simulink model "test_mosfet_dynamic"  (R2021b)
settings: Solver=VariableStepAuto  StartTime=0.0  StopTime=0.1  RelTol=1e-3
libraries: fl_lib x17, nesl_utility x12, ee_lib x5, simulink x1
settings Model: PauseTimes=0.1  Creator=khduh  LastModifiedBy=user
settings DataIOCC: SaveState=on
settings SimscapeCC: SimscapeLogType=all  SimscapeLogLimitData=off

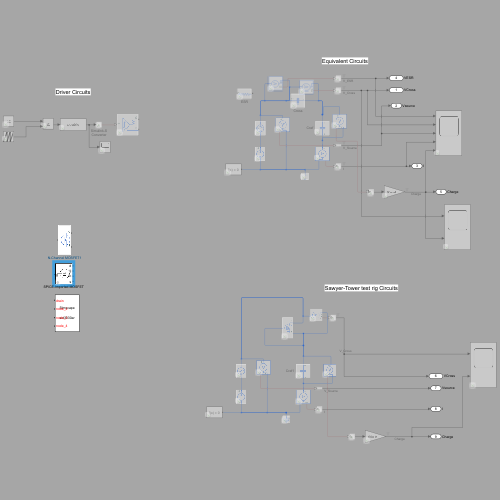
[thumbnail: Simulink's stored preview of the top-level diagram]
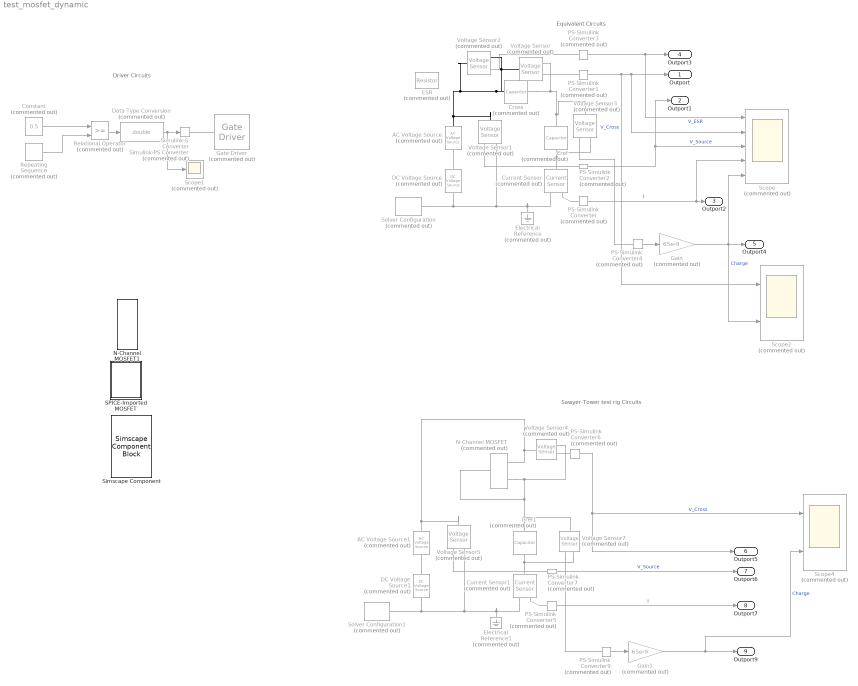
== system test_mosfet_dynamic ==
  note: Driver Circuits
  note: Equivalent Circuits
  note: Sawyer-Tower test rig Circuits
  AC Voltage Source : fl_lib/Electrical/Electrical Sources/AC Voltage Source  Commented=on  amp=50 V  shift=0 deg  frequency=60 Hz  omega=0 rad/s
  AC Voltage Source1 : fl_lib/Electrical/Electrical Sources/AC Voltage Source  Commented=on  amp=50 V  shift=0 deg  frequency=60 Hz  omega=0 rad/s
  Constant : Constant  Commented=on  Value=0.5
  Cref : fl_lib/Electrical/Electrical Elements/Capacitor  Commented=on  c=65e-9 F  r=1e-6 Ohm  g=0 1/Ohm  i_specify=off  i_priority=None  i=0 A  i_nominal_specify=off  i_nominal_unit=A  i_nominal_value=1  v_specify=off  v_priority=None  v=0 V  v_nominal_specify=off  v_nominal_unit=V  v_nominal_value=1  vc_specify=off  vc_priority=High  vc=0 V  vc_nominal_specify=off  vc_nominal_unit=V  vc_nominal_value=1
  Cref1 : fl_lib/Electrical/Electrical Elements/Capacitor  Commented=on  c=65e-9 F  r=1e-6 Ohm  g=0 1/Ohm  i_specify=off  i_priority=None  i=0 A  i_nominal_specify=off  i_nominal_unit=A  i_nominal_value=1  v_specify=off  v_priority=None  v=0 V  v_nominal_specify=off  v_nominal_unit=V  v_nominal_value=1  vc_specify=off  vc_priority=High  vc=0 V  vc_nominal_specify=off  vc_nominal_unit=V  vc_nominal_value=1
  Cross : fl_lib/Electrical/Electrical Elements/Capacitor  Commented=on  c=89e-9 F  r=1e-6 Ohm  g=0 1/Ohm  i_specify=off  i_priority=None  i=0 A  i_nominal_specify=off  i_nominal_unit=A  i_nominal_value=1  v_specify=off  v_priority=None  v=0 V  v_nominal_specify=off  v_nominal_unit=V  v_nominal_value=1  vc_specify=off  vc_priority=High  vc=0 V  vc_nominal_specify=off  vc_nominal_unit=V  vc_nominal_value=1
  Current Sensor : fl_lib/Electrical/Electrical Sensors/Current Sensor  Commented=on
  Current Sensor1 : fl_lib/Electrical/Electrical Sensors/Current Sensor  Commented=on
  DC Voltage Source : ee_lib/Additional Components/SPICE Sources/DC Voltage Source  Commented=on  DC=100 V
  DC Voltage Source1 : ee_lib/Additional Components/SPICE Sources/DC Voltage Source  Commented=on  DC=500 V
  Data Type Conversion : DataTypeConversion  Commented=on  OutDataTypeStr=double
  ESR : fl_lib/Electrical/Electrical Elements/Resistor  Commented=on  R=58.5e3 Ohm  i_specify=off  i_priority=None  i=0 A  i_nominal_specify=off  i_nominal_unit=A  i_nominal_value=1  v_specify=off  v_priority=None  v=0 V  v_nominal_specify=off  v_nominal_unit=V  v_nominal_value=1
  Electrical Reference : fl_lib/Electrical/Electrical Elements/Electrical Reference  Commented=on
  Electrical Reference1 : fl_lib/Electrical/Electrical Elements/Electrical Reference  Commented=on
  Gain : Gain  Commented=on  Gain=65e-9
  Gain1 : Gain  Commented=on  Gain=65e-9
  Gate Driver : ee_lib/Semiconductors & Converters/Gate Driver  Commented=on  uHighValue=0.7  uLowValue=0.3  vHigh=4 V  vLow=0 V  tHigh=50 ns  tLow=50 ns  parameterization=1  rHigh=2 Ohm  rLow=2 Ohm  tRise=20 ns  tFall=20 ns  cLoad=10 nF  enable_faults=0  t_fault=1 s  fault_type=1  ZonTime_specify=off  ZonTime_priority=None  ZonTime=0 s  ZoffTime_specify=off  ZoffTime_priority=None  ZoffTime=0 s  uHigh=2.0 V  uLow=0.8 V
      settings: SourceProductBaseCode=PS  InternalSimscapePortConfiguration="{\"Bottom\":[],\"Left\":[{\"id\":\"u\",\"label\":\"u\",\"type\":\"input\"}],\"Right\":[{\"id\":\"G\",\"label\":\"G\",\"type\":\"foundation.electrical.electrical\"},{\"id\":\"S\",\"label\":\"S\",\"type\":\"foundation.electrical.electrical\"}],\"Top\":[]}"
  N-Channel MOSFET : ee_lib/Semiconductors & Converters/N-Channel MOSFET  Commented=on  paramTerminal=ee.enum.mosfet.numberOfTerminals.three  parameterization=ee.enum.mosfet.parameterization.datasheet  Beta=5.0 A/V^2  Rds=0.025 Ohm  Id=6.0 A  Vgs=10 V  Vth=1.7 V  Vth0=1.7 V  lam=0 1/V  gamma_vth=0.5 V^(1/2)  phib=0.5 V  Vth1=1.9071 V  Vbs1=-1 V  Vth2=2.066 V  Vbs2=-2 V  Tmeas=25 degC  Vgs_vec=[-.5, 2, 3, 4, 5] V  Vds_vec=[0, 2, 4, 8, 12, 16, 20] V  Vbs_vec=[0, -4, -6, -12] V  T_vec=[25, 125] degC  Vth_vec=[.4, 1.2, 1.4, 1.45] V  Vth_mat=[.4, .35; 1.2, 1.15; 1.4, 1.35; 1.45, 1.4] V  Ids_mat=[0, 0, 0, 0, 0, 0, 0; 0, .003, .0038, .0043, .0046, .0048, .0049; 0, .0055, .008, .009, .0095, .01, .0101; 0, .0115, .016, .018, .019, .0195, .02; 0, .0152, .0225, .0265, .028, .0295, .03] A  Ids_mat0=[0, 0, 0, 0, 0, 0, 0; 0, .003, .0038, .0043, .0046, .0048, .0049; 0, .0055, .008, .009, .0095, .01, .0101; 0, .0115, .016, .018, .019, .0195, .02; 0, .0152, .0225, .0265, .028, .0295, .03] A  Ids_mat_3D=zeros(5, 7, 2) A  Ids_mat_3D0=zeros(5, 7, 2) A  IV_table_symmetry=ee.enum.mosfet.symmetricNIV.no  RS=0.0001 Ohm  RD=0.01 Ohm  RB=0.001 Ohm  C_param=ee.enum.mosfet.capacitanceParam.fixedciss  C_GS=270 pF  C_GD=80 pF  C_DS=0 pF  C_iss=1526 pF  C_rss=42 pF  C_oss=89 pF  charge_linearity_param=ee.enum.mosfet.cgdLinearity.constant  C_OX=200 pF  V_C_OX=-0.5 V  charge_linearity_param_vgb=ee.enum.mosfet.cgbLinearity.instantly  C_iss_vec=[720, 700, 590, 470, 390, 310] pF  C_rss_vec=[450, 400, 300, 190, 95, 55] pF  C_oss_vec=[900, 810, 690, 420, 270, 170] pF  C_GS_vec=[270, 300, 290, 280, 295, 255] pF  C_GD_vec=[450, 400, 300, 190, 95, 55] pF  C_DS_vec=[450, 410, 390, 230, 175, 115] pF  C_Vds_vec=[.1, .3, 1, 3, 10, 30] V  V_GS_for_cap_data=0 V  Di_param=ee.enum.mosfet.diodeParam.no  IsDiode=0 A  Vbi=0.6 V  n=1  Cj0Diode=0 pF  TT=50e-9 s  Tmeas_dio=25 degC  TableTypeNoT=ee.enum.mosfet.tableType.IfMat  TableType=ee.enum.diode.tableType.IfMat  IfVec=[.07, .12, .19, 1.75, 4.24, 7.32, 11.2] A  IfMat=[.07, .12, .19, 1.75, 4.24, 7.32, 11.2; .16, .3, .72, 2.14, 4.02, 6.35, 9.12] A  VfVecV=[.9, 1.15, 1.25, 1.5, 1.75, 2.17, 2.6, 2.85] V  VfMatV=[.9, 1.15, 1.25, 1.5, 1.75, 2.17, 2.6, 2.85; .58, .68, .75, 1.1, 1.38, 1.77, 2.27, 2.7] V  TjVec=[25, 125] degC  VfVec=[.5, .7, .9, 1.3, 1.7, 2.1, 2.5] V  IfVecV=[.1, .2, .5, 1, 2, 4, 7, 10] A  prmDatasheet=ee.enum.temperatureParameterization.none  prmEquCoeff=ee.enum.temperatureParameterization.none  dVth_dT=-6 mV/K  dVth0_dT=-6 mV/K  Rds_T2=0.037 Ohm  BEXDatasheet=-1.5  BEXEquCoeff=-1.5  etaisDatasheet=3  etaisEquCoeff=3  Tmeas2=125 degC  etaisTabulated=3  TdeviceDatasheet=25 degC  TdeviceEquCoeff=25 degC  TdeviceTabulated=25 degC  thermal_network_parameterization=ee.enum.thermalNetworkTopology.junctionCase  Rth=[0, 10] K/W  Rth_Cauer=[1, 3, 10] K/W  Rth_Foster=[4, 6] K/W  thermal_mass_parameterization=ee.enum.thermalNetwork.timeconstant  thermal_mass=[0, 1] J/K  thermal_mass_Cauer=[.1, .3, 1] J/K  thermal_mass_Foster=[1.5, 3] J/K  thermal_time_constant=[0, 10] s  thermal_time_constant_Cauer=[1, 3, 10] s  thermal_time_constant_Foster=[6, 18] s  thermal_mass_initial_temperatures=[25, 25] degC  thermal_mass_initial_temperatures_Cauer=[25, 25, 25] degC  steadyState_Foster=simscape.enum.onoff.on  Tvec_initial_Foster=[25, 25, 25, 25] degC  betaref=18 A/V^2  Vfbref=-1.1 V  gamma=3.5 V^(1/2)  phib2ref=1 V  thesatref=0.4 1/V  alpha=0  Vp=5e-2 V  thesrref=0 1/V  m=8  Tref=25 degC  Rsref=2e-3 Ohm  Rdref=0.17 Ohm  Rgref=8.4 Ohm  Rbref=2e-3 Ohm  Cox=1500 pF  Cgso=100 pF  Cgdo=14 pF  Isref=5.2e-13 A  Cj0=480 pF  Tprm=1  etabet=1.3  Stvfb=5e-4 V/K  Stphib=-8.5e-4 V/K  etasat=1.04  etasr=0.65  etar=0.95  etais=3  Tsim=25 degC  T0=[25, 25] degC  T0_Cauer=[25, 25, 25] degC
  N-Channel MOSFET1 : ee_lib/Semiconductors & Converters/N-Channel MOSFET  paramTerminal=ee.enum.mosfet.numberOfTerminals.three  parameterization=ee.enum.mosfet.parameterization.datasheet  Beta=5.0 A/V^2  Rds=0.025 Ohm  Id=6.0 A  Vgs=10 V  Vth=1.7 V  Vth0=1.7 V  lam=0 1/V  gamma_vth=0.5 V^(1/2)  phib=0.5 V  Vth1=1.9071 V  Vbs1=-1 V  Vth2=2.066 V  Vbs2=-2 V  Tmeas=25 degC  Vgs_vec=[-.5, 2, 3, 4, 5] V  Vds_vec=[0, 2, 4, 8, 12, 16, 20] V  Vbs_vec=[0, -4, -6, -12] V  T_vec=[25, 125] degC  Vth_vec=[.4, 1.2, 1.4, 1.45] V  Vth_mat=[.4, .35; 1.2, 1.15; 1.4, 1.35; 1.45, 1.4] V  Ids_mat=[0, 0, 0, 0, 0, 0, 0; 0, .003, .0038, .0043, .0046, .0048, .0049; 0, .0055, .008, .009, .0095, .01, .0101; 0, .0115, .016, .018, .019, .0195, .02; 0, .0152, .0225, .0265, .028, .0295, .03] A  Ids_mat0=[0, 0, 0, 0, 0, 0, 0; 0, .003, .0038, .0043, .0046, .0048, .0049; 0, .0055, .008, .009, .0095, .01, .0101; 0, .0115, .016, .018, .019, .0195, .02; 0, .0152, .0225, .0265, .028, .0295, .03] A  Ids_mat_3D=zeros(5, 7, 2) A  Ids_mat_3D0=zeros(5, 7, 2) A  IV_table_symmetry=ee.enum.mosfet.symmetricNIV.no  RS=0.0001 Ohm  RD=0.01 Ohm  RB=0.001 Ohm  C_param=ee.enum.mosfet.capacitanceParam.fixedciss  C_GS=270 pF  C_GD=80 pF  C_DS=0 pF  C_iss=350 pF  C_rss=80 pF  C_oss=0 pF  charge_linearity_param=ee.enum.mosfet.cgdLinearity.constant  C_OX=200 pF  V_C_OX=-0.5 V  charge_linearity_param_vgb=ee.enum.mosfet.cgbLinearity.instantly  C_iss_vec=[720, 700, 590, 470, 390, 310] pF  C_rss_vec=[450, 400, 300, 190, 95, 55] pF  C_oss_vec=[900, 810, 690, 420, 270, 170] pF  C_GS_vec=[270, 300, 290, 280, 295, 255] pF  C_GD_vec=[450, 400, 300, 190, 95, 55] pF  C_DS_vec=[450, 410, 390, 230, 175, 115] pF  C_Vds_vec=[.1, .3, 1, 3, 10, 30] V  V_GS_for_cap_data=0 V  Di_param=ee.enum.mosfet.diodeParam.no  IsDiode=0 A  Vbi=0.6 V  n=1  Cj0Diode=0 pF  TT=50e-9 s  Tmeas_dio=25 degC  TableTypeNoT=ee.enum.mosfet.tableType.IfMat  TableType=ee.enum.diode.tableType.IfMat  IfVec=[.07, .12, .19, 1.75, 4.24, 7.32, 11.2] A  IfMat=[.07, .12, .19, 1.75, 4.24, 7.32, 11.2; .16, .3, .72, 2.14, 4.02, 6.35, 9.12] A  VfVecV=[.9, 1.15, 1.25, 1.5, 1.75, 2.17, 2.6, 2.85] V  VfMatV=[.9, 1.15, 1.25, 1.5, 1.75, 2.17, 2.6, 2.85; .58, .68, .75, 1.1, 1.38, 1.77, 2.27, 2.7] V  TjVec=[25, 125] degC  VfVec=[.5, .7, .9, 1.3, 1.7, 2.1, 2.5] V  IfVecV=[.1, .2, .5, 1, 2, 4, 7, 10] A  prmDatasheet=ee.enum.temperatureParameterization.none  prmEquCoeff=ee.enum.temperatureParameterization.none  dVth_dT=-6 mV/K  dVth0_dT=-6 mV/K  Rds_T2=0.037 Ohm  BEXDatasheet=-1.5  BEXEquCoeff=-1.5  etaisDatasheet=3  etaisEquCoeff=3  Tmeas2=125 degC  etaisTabulated=3  TdeviceDatasheet=25 degC  TdeviceEquCoeff=25 degC  TdeviceTabulated=25 degC  thermal_network_parameterization=ee.enum.thermalNetworkTopology.junctionCase  Rth=[0, 10] K/W  Rth_Cauer=[1, 3, 10] K/W  Rth_Foster=[4, 6] K/W  thermal_mass_parameterization=ee.enum.thermalNetwork.timeconstant  thermal_mass=[0, 1] J/K  thermal_mass_Cauer=[.1, .3, 1] J/K  thermal_mass_Foster=[1.5, 3] J/K  thermal_time_constant=[0, 10] s  thermal_time_constant_Cauer=[1, 3, 10] s  thermal_time_constant_Foster=[6, 18] s  thermal_mass_initial_temperatures=[25, 25] degC  thermal_mass_initial_temperatures_Cauer=[25, 25, 25] degC  steadyState_Foster=simscape.enum.onoff.on  Tvec_initial_Foster=[25, 25, 25, 25] degC  betaref=18 A/V^2  Vfbref=-1.1 V  gamma=3.5 V^(1/2)  phib2ref=1 V  thesatref=0.4 1/V  alpha=0  Vp=5e-2 V  thesrref=0 1/V  m=8  Tref=25 degC  Rsref=2e-3 Ohm  Rdref=0.17 Ohm  Rgref=8.4 Ohm  Rbref=2e-3 Ohm  Cox=1500 pF  Cgso=100 pF  Cgdo=14 pF  Isref=5.2e-13 A  Cj0=480 pF  Tprm=1  etabet=1.3  Stvfb=5e-4 V/K  Stphib=-8.5e-4 V/K  etasat=1.04  etasr=0.65  etar=0.95  etais=3  Tsim=25 degC  T0=[25, 25] degC  T0_Cauer=[25, 25, 25] degC
  PS-Simulink Converter{,1..7,9} (9 alike) : nesl_utility/PS-Simulink Converter  Commented=on  PhysicalDomain=network_engine_domain  SubClassName=ps_output  LeftPortType=input  RightPortType=output  PseudoPeriodic=off  Frequencies=[]  Unit=inherit  AffineConversion=off
      settings: SourceProductBaseCode=PW,SS
  Relational Operator : RelationalOperator  Commented=on  OutDataTypeStr=boolean  RndMeth=Simplest
  Repeating Sequence : simulink/Sources/Repeating Sequence  Commented=on  rep_seq_t=[0 100e-6]  rep_seq_y=[0 1]
  SPICE-Imported MOSFET : Subsystem  mask(SPICE-Imported MOSFET){SeriesChoice=Infineon OptiMOS6 40V, DeviceOptiMOS40V=IAUC120N04S6N009, DeviceOptiMOS60V=IPB120N06S4_H1, DeviceOptiMOS80V=IAUT300N08S5N012, DeviceOptiMOS120V=IPB100N12S3_05}
      mask prompts: SeriesChoice "Series"; DeviceOptiMOS40V "Device"; DeviceOptiMOS60V "Device"; DeviceOptiMOS80V "Device"; DeviceOptiMOS120V "Device"
      mask help: MOSFET model converted from SPICE.<br/> <br/> To view information pertaining to this device model, see the <a href="matlab: ee.internal.spice.openAndGoToLine('Infineon-OptiMOS6_40V-SimulationModels-v02_00-EN.lib','IAUC120N04S6N009')">originating SPICE file</a>.
      mask init:
      | ee.internal.spice.maskCallbackMOSFETs(gcb)
      settings: CopyFcn=set_param(gcb,'LinkStatus','none');
      mask Help: web(nesl_help(gcbh))
      mask TypeOptions SeriesChoice: Infineon OptiMOS6 40V | Infineon OptiMOS4 60V | Infineon OptiMOS5 80V | Infineon OptiMOST 120V
      mask Callback SeriesChoice:
      | %Run mask initialization to update the block help
      | ee.internal.spice.maskCallbackMOSFETs(gcb)
      mask TypeOptions DeviceOptiMOS40V: IAUC120N04S6N009 | IAUC120N04S6N010 | IAUC120N04S6N013 | IAUC100N04S6N015 | IAUC100N04S6N022 | IAUC100N04S6N028 | IAUC80N04S6N036 | IAUC60N04S6N044 | IAUC120N04S6L008 | IAUC120N04S6L009 | IAUC120N04S6L012 | IAUC100N04S6L014 | IAUC100N04S6L020 | IAUC100N04S6L025 | IAUC80N04S6L032 | IAUC60N04S6L039
      mask Callback DeviceOptiMOS40V:
      | %Run mask initialization to update the block help
      | ee.internal.spice.maskCallbackMOSFETs(gcb)
      mask TypeOptions DeviceOptiMOS60V: IPB180N06S4_H1 | IPB120N06S4_H1 | IPI120N06S4_H1 | IPP120N06S4_H1 | IPB120N06S4_02 | IPI120N06S4_02 | IPP120N06S4_02 | IPB120N06S4_03 | IPI120N06S4_03 | IPP120N06S4_03 | IPB90N06S4_04 | IPD90N06S4_04 | IPD100N06S4_03 | IPI90N06S4_04 | IPP90N06S4_04 | IPB80N06S4_05 | IPD90N06S4_05 | IPI80N06S4_05 | IPP80N06S4_05 | IPB80N06S4_07 | IPD90N06S4_07 | IPI80N06S4_07 | IPP80N06S4_07 | IPB45N06S4_09 | IPD50N06S4_09 | IPI45N06S4_09 | IPP45N06S4_09 | IPG20N06S4_15 | IPB90N06S4L_04 | IPD90N06S4L_03 | IPI90N06S4L_04 | IPP90N06S4L_04 | IPB80N06S4L_05 | IPD90N06S4L_05 | IPI80N06S4L_05 | IPP80N06S4L_05 | IPB80N06S4L_07 | IPD90N06S4L_06 | IPI80N06S4L_07 | IPP80N06S4L_07 | IPB45N06S4L_08 | IPD50N06S4L_08 | IPI45N06S4L_08 | IPP45N06S4L_08 | IPD50N06S4L_12 | IPD30N06S4L_23 | IPD25N06S4L_30 | IPG20N06S4L_11 | IPG20N06S4L_14 | IPG20N06S4L_26
      mask Callback DeviceOptiMOS60V:
      | %Run mask initialization to update the block help
      | ee.internal.spice.maskCallbackMOSFETs(gcb)
      mask TypeOptions DeviceOptiMOS80V: IPB015N08N5 | IPB017N08N5 | IPP020N08N5 | IPT012N08N5 | IPB020N08N5 | IPP023N08N5 | IPB024N08N5 | IPP027N08N5 | IPB031N08N5 | IPP034N08N5 | IPB049N08N5 | IPP052N08N5 | IAUT300N08S5N012 | IAUT165N08S5N029 | IAUT300N08S5N014 | IAUT240N08S5N019 | IAUT200N08S5N023 | IAUS300N08S5N013T | IAUS300N08S5N015T | IAUC100N08S5N031 | IAUC100N08S5N043 | IAUC70N08S5N074
      mask Callback DeviceOptiMOS80V:
      | %Run mask initialization to update the block help
      | ee.internal.spice.maskCallbackMOSFETs(gcb)
      mask TypeOptions DeviceOptiMOS120V: IPB100N12S3_05 | IPI100N12S3_05 | IPP100N12S3_05 | IPB70N12S3_11 | IPI70N12S3_11 | IPP70N12S3_11 | IPD70N12S3_11 | IPD70N12S3L_12 | IPB70N12S3L_12 | IPI70N12S3L_12 | IPP70N12S3L_12 | IPB50N12S3L_15 | IPD50N12S3L_15 | IPI50N12S3L_15 | IPP50N12S3L_15 | IPB35N12S3L_26 | IPD35N12S3L_24 | IPD30N12S3L_31
      mask Callback DeviceOptiMOS120V:
      | %Run mask initialization to update the block help
      | ee.internal.spice.maskCallbackMOSFETs(gcb)
      mask DialogControl ParameterGroupVar Prompt: Device selection
  Scope : Scope  Commented=on  NumInputPorts=5
  Scope1 : Scope  Commented=on
  Scope2 : Scope  Commented=on  NumInputPorts=2
  Scope4 : Scope  Commented=on  NumInputPorts=2
  Simscape Component : SimscapeComponentBlock  SourceFile=myLIB.sct3030ar  ComponentPath=myLIB.sct3030ar  ComponentVariants="[\"myLIB.sct3030ar\"]"  ComponentVariantNames="[\"sct3030ar\"]"  ClassName=sct3030ar  SchemaVersion=1  temp=27  specifyParasiticValues=ee.enum.include.no  capacitorSeriesResistance=0 Ohm  inductorParallelConductance=0 1/Ohm  specifySmoothValues=ee.enum.include.no  aWarning=ee.enum.include.no  crossZero=ee.enum.include.no  dropPowerFlag=ee.enum.function.powerFlag.hyp  dropPowerHypEpsilon=0  expXh=Inf  expXl=-Inf  hyperbolicMaximumAbsolute=Inf  smoothEpsilon=0  smoothN=1  E1_specify=off  E1_priority=None  E1=0 A  E1_nominal_specify=off  E1_nominal_unit=A  E1_nominal_value=1  E2_specify=off  E2_priority=None  E2=0 A  E2_nominal_specify=off  E2_nominal_unit=A  E2_nominal_value=1  E6_specify=off  E6_priority=None  E6=0 A  E6_nominal_specify=off  E6_nominal_unit=A  E6_nominal_value=1  E7_specify=off  E7_priority=None  E7=0 A  E7_nominal_specify=off  E7_nominal_unit=A  E7_nominal_value=1  G6_specify=off  G6_priority=None  G6=0 A  G6_nominal_specify=off  G6_nominal_unit=A  G6_nominal_value=1  G1_specify=off  G1_priority=None  G1=0 A  G1_nominal_specify=off  G1_nominal_unit=A  G1_nominal_value=1  G2_specify=off  G2_priority=None  G2=0 A  G2_nominal_specify=off  G2_nominal_unit=A  G2_nominal_value=1  E11_specify=off  E11_priority=None  E11=0 A  E11_nominal_specify=off  E11_nominal_unit=A  E11_nominal_value=1  G11_specify=off  G11_priority=None  G11=0 A  G11_nominal_specify=off  G11_nominal_unit=A  G11_nominal_value=1
      settings: CopyFcn=simscape.engine.sli.internal.componentblockcallback(gcbh,'COPY')  PreCopyFcn=simscape.engine.sli.internal.componentblockcallback(gcbh,'PRECOPY')  PreDeleteFcn=simscape.engine.sli.internal.componentblockcallback(gcbh,'PREDELETE')  InternalSimscapePortConfiguration="{\"Bottom\":[],\"Left\":[{\"id\":\"node_1\",\"label\":\"drain\",\"type\":\"foundation.electrical.electrical\"},{\"id\":\"node_2\",\"label\":\"node_2\",\"type\":\"foundation.electrical.electrical\"},{\"id\":\"node_3\",\"label\":\"node_3\",\"type\":\"foundation.electrical.electrical\"},{\"id\":\"node_4\",\"label\":\"node_4\",\"type\":\"foundation.electrical.electrical\"}],\"Right\":[],\"Top\":[]}"
      mask Type: sct3030ar
  Simulink-S Converter : nesl_utility/Simulink-PS Converter  Commented=on  PhysicalDomain=network_engine_domain  SubClassName=ps_input  LeftPortType=input  RightPortType=output  PseudoPeriodic=off  Frequencies=[]  NoiseDistribution=none  NoiseParameters=[]  Unit=1  AffineConversion=off  FilteringAndDerivatives=provide  SimscapeFilterOrder=1  InputFilterTimeConstant=0.001  UdotUserProvided=0
      settings: SourceProductBaseCode=PW,SS
  Solver Configuration : nesl_utility/Solver Configuration  Commented=on  PhysicalDomain=network_engine_domain  SubClassName=solver  LeftPortType=input  RightPortType=generic  Tones=[]  Harmonics=[]  SimulateNoise=off  Profile=off  UseLocalSampling=off  EnableSwitchedLinearOptims=on  FrequencyDomain=off  UseCCode=off  RelTol=0.001  AbsTol=1e-06  MinStep=1e-09  ToWorkspace=off  RevertToSquareIcSolve=off  NumHomotopyIterations=100  PhasorMode=off  PhasorModeNumHarmonics=1  DoDC=off  ResidualTolerance=1e-09  UseLocalSolver=off  LocalSolverChoice=NE_BACKWARD_EULER_ADVANCER  LocalSolverSampleTime=0.001  DoFixedCost=off  MaxNonlinIter=3  MaxModeIter=2  ComputeImpulses=off  ImpulseIterations=2  LinearAlgebra=auto  EquationFormulation=NE_TIME_EF  DelaysMemoryBudget=1024  AutomaticFiltering=on  FilteringTimeConstant=0.001  PartitionStorageMethod=AS_NEEDED  PartitionMemoryBudget=1024  PartitionMethod=ROBUST
      settings: SourceProductBaseCode=PW,SS
  Solver Configuration1 : nesl_utility/Solver Configuration  Commented=on  PhysicalDomain=network_engine_domain  SubClassName=solver  LeftPortType=input  RightPortType=generic  Tones=[]  Harmonics=[]  SimulateNoise=off  Profile=off  UseLocalSampling=off  EnableSwitchedLinearOptims=on  FrequencyDomain=off  UseCCode=off  RelTol=0.001  AbsTol=1e-06  MinStep=1e-09  ToWorkspace=off  RevertToSquareIcSolve=off  NumHomotopyIterations=100  PhasorMode=off  PhasorModeNumHarmonics=1  DoDC=off  ResidualTolerance=1e-09  UseLocalSolver=off  LocalSolverChoice=NE_BACKWARD_EULER_ADVANCER  LocalSolverSampleTime=0.001  DoFixedCost=off  MaxNonlinIter=3  MaxModeIter=2  ComputeImpulses=off  ImpulseIterations=2  LinearAlgebra=auto  EquationFormulation=NE_TIME_EF  DelaysMemoryBudget=1024  AutomaticFiltering=on  FilteringTimeConstant=0.001  PartitionStorageMethod=AS_NEEDED  PartitionMemoryBudget=1024  PartitionMethod=ROBUST
      settings: SourceProductBaseCode=PW,SS
  Voltage Sensor{,1..5,7} (7 alike) : fl_lib/Electrical/Electrical Sensors/Voltage Sensor  Commented=on
  Outport : Outport  SignalName=VCross
  Outport1 : Outport  Port=2  SignalName=Vsource
  Outport2 : Outport  Port=3  SignalName=I
  Outport3 : Outport  Port=4  SignalName=VESR
  Outport4 : Outport  Port=5  SignalName=Charge
  Outport5 : Outport  Port=6  SignalName=VCross
  Outport6 : Outport  Port=7  SignalName=Vsource
  Outport7 : Outport  Port=8  SignalName=I
  Outport9 : Outport  Port=9  SignalName=Charge
  wires:
  PS-Simulink Converter/1 -> Scope/4, Outport2/1  "I"
  Repeating Sequence/1 -> Relational Operator/2
  Constant/1 -> Relational Operator/1
  Relational Operator/1 -> Data Type Conversion/1
  Data Type Conversion/1 -> Simulink-S Converter/1, Scope1/1
  PS-Simulink Converter1/1 -> Scope2/1, Outport/1, Scope/2  "V_Cross"
  PS-Simulink Converter2/1 -> Outport1/1, Scope/3  "V_Source"
  PS-Simulink Converter3/1 -> Scope/1, Outport3/1  "V_ESR"
  PS-Simulink Converter4/1 -> Gain/1
  Gain/1 -> Scope/5, Outport4/1, Scope2/2  "Charge"
  PS-Simulink Converter9/1 -> Gain1/1
  Gain1/1 -> Outport9/1, Scope4/2  "Charge"
  PS-Simulink Converter7/1 -> Outport6/1  "V_Source"
  PS-Simulink Converter6/1 -> Outport5/1, Scope4/1  "V_Cross"
  PS-Simulink Converter5/1 -> Outport7/1  "I"
  connections:
  Electrical Reference/LConn1 -- DC Voltage Source/RConn1 -- Solver Configuration/RConn1 -- Voltage Sensor1/RConn2 -- Current Sensor/RConn2
  PS-Simulink Converter/LConn1 -- Current Sensor/RConn1
  Gate Driver/LConn1 -- Simulink-S Converter/RConn1
  DC Voltage Source/LConn1 -- AC Voltage Source/RConn1
  Cref/RConn1 -- Voltage Sensor3/RConn2 -- Current Sensor/LConn1
  AC Voltage Source/LConn1 -- Voltage Sensor2/RConn2 -- Voltage Sensor/LConn1 -- Cross/LConn1 -- Voltage Sensor2/LConn1 -- Voltage Sensor1/LConn1
  Cross/RConn1 -- Voltage Sensor/RConn2 -- Voltage Sensor3/LConn1 -- Cref/LConn1
  PS-Simulink Converter1/LConn1 -- Voltage Sensor/RConn1
  Voltage Sensor1/RConn1 -- PS-Simulink Converter2/LConn1
  PS-Simulink Converter3/LConn1 -- Voltage Sensor2/RConn1
  Voltage Sensor3/RConn1 -- PS-Simulink Converter4/LConn1
  AC Voltage Source1/LConn1 -- N-Channel MOSFET/RConn1 -- Voltage Sensor4/LConn1 -- Voltage Sensor5/LConn1
  Solver Configuration1/RConn1 -- Voltage Sensor5/RConn2 -- Electrical Reference1/LConn1 -- Current Sensor1/RConn2 -- DC Voltage Source1/RConn1
  Cref1/RConn1 -- Voltage Sensor7/RConn2 -- Current Sensor1/LConn1
  Voltage Sensor5/RConn1 -- PS-Simulink Converter7/LConn1
  DC Voltage Source1/LConn1 -- AC Voltage Source1/RConn1
  PS-Simulink Converter5/LConn1 -- Current Sensor1/RConn1
  Voltage Sensor7/RConn1 -- PS-Simulink Converter9/LConn1
  Cref1/LConn1 -- Voltage Sensor7/LConn1 -- N-Channel MOSFET/LConn1 -- N-Channel MOSFET/RConn2 -- Voltage Sensor4/RConn2
  Voltage Sensor4/RConn1 -- PS-Simulink Converter6/LConn1

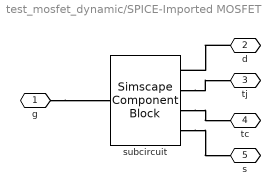
== system test_mosfet_dynamic/SPICE-Imported MOSFET ==
  subcircuit : SimscapeComponentBlock  SourceFile=ee_spice_mosfets.spiceinfineon.spiceOptiMOS_6_40V.IAUC120N04S6N009_wrapped  ComponentPath=ee_spice_mosfets.spiceinfineon.spiceOptiMOS_6_40V.IAUC120N04S6N009_wrapped  ComponentVariants="[\"ee_spice_mosfets.spiceinfineon.spiceOptiMOS_6_40V.IAUC120N04S6N009_wrapped\"]"  ComponentVariantNames="[\"IAUC120N04S6N009_wrapped\"]"  ClassName=IAUC120N04S6N009_wrapped  SchemaVersion=1
      settings: CopyFcn=simscape.engine.sli.internal.componentblockcallback(gcbh,'COPY')  PreCopyFcn=simscape.engine.sli.internal.componentblockcallback(gcbh,'PRECOPY')  PreDeleteFcn=simscape.engine.sli.internal.componentblockcallback(gcbh,'PREDELETE')  InternalSimscapePortConfiguration="{\"Bottom\":[],\"Left\":[{\"id\":\"gate\",\"label\":\"g\",\"type\":\"foundation.electrical.electrical\"}],\"Right\":[{\"id\":\"drain\",\"label\":\"d\",\"type\":\"foundation.electrical.electrical\"},{\"id\":\"tj\",\"label\":\"tj\",\"type\":\"foundation.electrical.electrical\"},{\"id\":\"tcase\",\"label\":\"tc\",\"type\":\"foundation.electrical.electrical\"},{\"id\":\"source\",\"label\":\"s\",\"type\":\"foundation.electrical.electrical\"}],\"Top\":[]}"
      mask Type: Infineon IAUC120N04S6N009
  g : PMIOPort  Side=Left
  d : PMIOPort  Port=2  Side=Right
  tj : PMIOPort  Port=3  Side=Right
  tc : PMIOPort  Port=4  Side=Right
  s : PMIOPort  Port=5  Side=Right
  connections:
  subcircuit/RConn4 -- s/RConn1
  subcircuit/RConn3 -- tc/RConn1
  subcircuit/RConn2 -- tj/RConn1
  d/RConn1 -- subcircuit/RConn1
  g/RConn1 -- subcircuit/LConn1
